simulink model "data"  (Simulink 8.3)
settings: Solver=ode45  StartTime=0.0  StopTime=simu_time  RelTol=1e-3
values from neighbouring files (symbols this model uses):
  Ex = 10^(0.1*SNR_Current)    (= 0.316227766017)    [main.m]
  Frame_Len = 4096    [Search_OrthogonalMatrix.m]    (also in main.m = 1024)
  K_ChannelDim = 128    [Search_OrthogonalMatrix.m]    (also in main.m = 64)
  pho = 0.2    [Search_OrthogonalMatrix.m]    (also in main.m)
  Sample_time = 1    [Search_OrthogonalMatrix.m]    (also in main.m)
libraries: commdigbbndpm3 x4, commrandsrc2 x2, commsink2 x2
settings Model: Creator=Administrator  LastModifiedBy=QCJ
settings DataIOCC: SignalLoggingSaveFormat=Dataset
settings DebuggingCC: UnderspecifiedInitializationDetection=Simplified  StateNameClashWarn=none
settings GRTTargetCC: CombineOutputUpdateFcns=on  GRTInterface=off

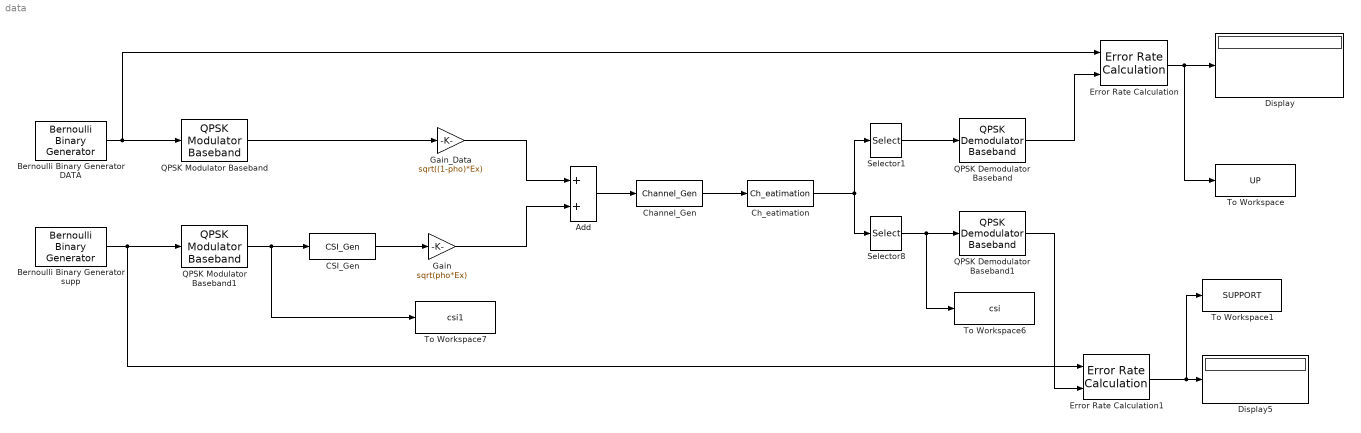
== system data ==
  Add : Sum
  "Bernoulli Binary Generator DATA " : commrandsrc2/Bernoulli Binary Generator  P=0.5  seed=61  Ts=Sample_time  frameBased=on  sampPerFrame=Frame_Len*2  orient=off  outDataType=double
  Bernoulli Binary Generator supp : commrandsrc2/Bernoulli Binary Generator  P=0.5  seed=61  Ts=Sample_time  frameBased=on  sampPerFrame=K_ChannelDim*2  orient=off  outDataType=double
  CSI_Gen : MATLABFcn  MATLABFcn=CSI_Gen  OutputSignalType=complex  Output1D=off
  Ch_eatimation : MATLABFcn  MATLABFcn=Ch_eatimation  OutputSignalType=complex  Output1D=off
  Channel_Gen : MATLABFcn  MATLABFcn=Channel_Gen  OutputSignalType=complex  Output1D=off
  Display : Display
  Display5 : Display
  Error Rate Calculation : commsink2/Error Rate Calculation  N=0  st_delay=0  cp_mode=Entire frame  subframe=[]  PMode=Port  WsName=ErrorVec  RsMode2=off  stop=off  numErr=100  maxBits=1e6
  Error Rate Calculation1 : commsink2/Error Rate Calculation  N=0  st_delay=0  cp_mode=Entire frame  subframe=[]  PMode=Port  WsName=ErrorVec  RsMode2=off  stop=off  numErr=100  maxBits=1e6
  Gain : Gain  Gain=sqrt(pho*Ex)
  Gain_Data : Gain  Gain=sqrt((1-pho)*Ex)
  QPSK Demodulator Baseband : commdigbbndpm3/QPSK Demodulator Baseband  Ph=pi/4  Dec=Gray  OutType=Bit  DecType=Hard decision  VarSource=Dialog  Variance=1  outDtype1=Inherit via internal rule  outDtype2=Inherit via internal rule  derotateFactorWordLen=16
  QPSK Demodulator Baseband1 : commdigbbndpm3/QPSK Demodulator Baseband  Ph=pi/4  Dec=Gray  OutType=Bit  DecType=Hard decision  VarSource=Dialog  Variance=1  outDtype1=Inherit via internal rule  outDtype2=Inherit via internal rule  derotateFactorWordLen=16
  QPSK Modulator Baseband : commdigbbndpm3/QPSK Modulator Baseband  InType=Bit  Enc=Gray  Ph=pi/4  outDtype=double  outWordLen=16  outUDDataType=sfix(16)  outFracLenMode=Best precision  outFracLen=15
  QPSK Modulator Baseband1 : commdigbbndpm3/QPSK Modulator Baseband  InType=Bit  Enc=Gray  Ph=pi/4  outDtype=double  outWordLen=16  outUDDataType=sfix(16)  outFracLenMode=Best precision  outFracLen=15
  Selector1 : Selector  InputPortWidth=K_ChannelDim + Frame_Len  Indices="[K_ChannelDim+1:K_ChannelDim  + Frame_Len]"
  Selector8 : Selector  InputPortWidth=K_ChannelDim + Frame_Len  Indices=[1:K_ChannelDim]
  To Workspace : ToWorkspace  VariableName=UP  SampleTime=-1
  To Workspace1 : ToWorkspace  VariableName=SUPPORT  SampleTime=-1
  To Workspace6 : ToWorkspace  VariableName=csi  SampleTime=-1
  To Workspace7 : ToWorkspace  VariableName=csi1  SampleTime=-1
  wires:
  "Bernoulli Binary Generator DATA "/1 -> Error Rate Calculation/1, QPSK Modulator Baseband/1
  QPSK Modulator Baseband/1 -> Gain_Data/1
  Gain_Data/1 -> Add/1
  Gain/1 -> Add/2
  QPSK Modulator Baseband1/1 -> To Workspace7/1, CSI_Gen/1
  CSI_Gen/1 -> Gain/1
  Add/1 -> Channel_Gen/1
  Channel_Gen/1 -> Ch_eatimation/1
  Ch_eatimation/1 -> Selector1/1, Selector8/1
  Selector1/1 -> QPSK Demodulator Baseband/1
  QPSK Demodulator Baseband/1 -> Error Rate Calculation/2
  Error Rate Calculation/1 -> To Workspace/1, Display/1
  Bernoulli Binary Generator supp/1 -> Error Rate Calculation1/1, QPSK Modulator Baseband1/1
  QPSK Demodulator Baseband1/1 -> Error Rate Calculation1/2
  Error Rate Calculation1/1 -> To Workspace1/1, Display5/1
  Selector8/1 -> To Workspace6/1, QPSK Demodulator Baseband1/1
